simulink model "PubIfDecisionLSM_MDL"  (R2020b)
settings: configuration reference "DspaceConfig" (kept outside this file)
PostLoadFcn:
  | if any(exist('dsrtsu_mdlpostloadfcn', 'file') ~= 0), dsrtsu_mdlpostloadfcn('Execute', bdroot); end
InitFcn:
  | , if any(exist('rtifpga_mdlclblib', 'file') ~= 0), rtifpga_mdlclblib('Init', bdroot); end,
  | , if any(exist('dsmpb_private', 'file') ~= 0), dsmpb_private('dsmpb_mdlclblib', 'Init', bdroot); end,
values from neighbouring files (symbols this model uses):
  P_LSM_ALC_Enable = 0.0    [LSM_Parameter.sldd]
  P_LSM_AwayEdge_offset = 0.1    [LSM_Parameter.sldd]
  P_LSM_CentValidErr = 1.0    [LSM_Parameter.sldd]
  P_LSM_DOP_C0_EN_Limit = 0.8    [LSM_Parameter.sldd]
  P_LSM_DOP_C0_out_Limit = 2.0    [LSM_Parameter.sldd]
  P_LSM_DOP_C1_EN_Limit : value not decoded    [LSM_Parameter.sldd]
  P_LSM_DOP_C1_out_Limit : value not decoded    [LSM_Parameter.sldd]
  P_LSM_DOP_C1AndC2_Lim_X : value not decoded    [LSM_Parameter.sldd]
  P_LSM_DOP_C2_EN_Limit : value not decoded    [LSM_Parameter.sldd]
  P_LSM_DOP_C2_out_Limit : value not decoded    [LSM_Parameter.sldd]
  P_LSM_DOP_In_Pre2Dop_Dis = 1.0    [LSM_Parameter.sldd]
  P_LSM_DOP_Out_Pre2Dop_Dis = 2.0    [LSM_Parameter.sldd]
  P_LSM_DOP_PreDis_X : value not decoded    [LSM_Parameter.sldd]
  P_LSM_DOP_PreDis_Y : value not decoded    [LSM_Parameter.sldd]
  P_LSM_DOPEnableSW = 1.0    [LSM_Parameter.sldd]
  P_LSM_DOPValid_CheckTime = 0.06    [LSM_Parameter.sldd]
  P_LSM_DoubleLine_Curr2Cent_Dislimit = 0.5    [LSM_Parameter.sldd]
  P_LSM_DoubleLine_Dop2Cent_Dislimit = 0.5    [LSM_Parameter.sldd]
  P_LSM_DoubleLine_DOPOut_C1 : value not decoded    [LSM_Parameter.sldd]
  P_LSM_DoubleLine_Pre2Cent_Dislimit = 1.0    [LSM_Parameter.sldd]
  P_LSM_Error_Limit = 0.5    [LSM_Parameter.sldd]
  P_LSM_IFV2CenterAxis = 0.0    [LSM_Parameter.sldd]
  P_LSM_IFV2RearAxis = 0.0    [LSM_Parameter.sldd]
  P_LSM_Line2Edge_limit = 0.5    [LSM_Parameter.sldd]
  P_LSM_Line_Error = 0.1    [LSM_Parameter.sldd]
  P_LSM_LineSTD_Limit = 0.15    [LSM_Parameter.sldd]
  P_LSM_NOH_Switch = 0.0    [LSM_Parameter.sldd]
  P_LSM_OTL_C0_Factor = 1.0    [LSM_Parameter.sldd]
  P_LSM_OTL_C1_Factor = 0.5    [LSM_Parameter.sldd]
  P_LSM_OTL_C2_Factor = 0.5    [LSM_Parameter.sldd]
  P_LSM_Pre2OnlyLineDis = 5.0    [LSM_Parameter.sldd]
  P_LSM_Pre_t = 0.0    [LSM_Parameter.sldd]
  P_LSM_SingleLine_Cent2Edge_Dislimit = 100.0    [LSM_Parameter.sldd]
  P_LSM_SingleLine_Curr2Cent_Dislimit = 0.2    [LSM_Parameter.sldd]
  P_LSM_SingleLine_Dop2Cent_Dislimit = 0.2    [LSM_Parameter.sldd]
  P_LSM_SingleLine_DOPOut_C1 : value not decoded    [LSM_Parameter.sldd]
  P_LSM_SingleLine_Pre2Cent_Dislimit = 0.5    [LSM_Parameter.sldd]
  P_LSM_TJALimitSpd = 60.0    [LSM_Parameter.sldd]
undefined symbols (not defined in the file or in its folder): P_lCS_IFV2CenterAxis, P_LCS_IFV2RearAxis, P_LSM_EntryEdge_offset, P_LSM_EntryLnChngEnSwitch, P_LSM_EntryVanishDis, P_LSM_LinetLostTime, P_LSM_LineWijCal_C12, P_LSM_LineWijCal_C13, P_LSM_MapValid_ErrorSwitch, P_LSM_PosLineLcFac, P_LSM_SpdLim_Stub_Spd, P_LSM_SpdLim_StubLength, P_LSM_SpdTurnAlarm
libraries: simulink x324, TrueDurationTime x11
(part 16 of 25)

== stateflow chart PubIfDecisionLSM_MDL/Subsystem1/TargetLineCalc_20ms/TargetLineCalc/Subsystem3/Subsystem/Chart1 ==
  state on
    state CruiseValid2
      PilotRoadSts=18;
      LSM_PilotSPL=uint8(60);
      PilotSPLDist=uint16(0);
      state init
        state Name
          PilotTurnSwSts =0;
        state init4
          PilotTurnSwSts =6;
        state init5
          PilotTurnSwSts =3;
        state init3
          PilotTurnSwSts =7;
        (default) -> on.CruiseValid2.init.Name
        on.CruiseValid2.init.Name -> on.CruiseValid2.init.init3 [order 3] : [FrbRight>0]
        on.CruiseValid2.init.init3 -> on.CruiseValid2.init.Name : [FrbRight==0]
        on.CruiseValid2.init.Name -> on.CruiseValid2.init.init4 [order 1] : [FrbLeft>0]
        on.CruiseValid2.init.init4 -> on.CruiseValid2.init.Name : [FrbLeft==0]
        on.CruiseValid2.init.Name -> on.CruiseValid2.init.init5 [order 2] : [OneLane>0]
        on.CruiseValid2.init.init5 -> on.CruiseValid2.init.Name : [OneLane==0]
      state Name2
        PilotTurnSwSts=1;
      state init1
        PilotTurnSwSts =1;
      state init2
        PilotTurnSwSts =2;
      (default) -> on.CruiseValid2.init
      on.CruiseValid2.init -> on.CruiseValid2.Name2 [order 1] : [Vanish_turnleft>0]
      on.CruiseValid2.Name2 -> on.CruiseValid2.init : [Vanish_turnleft==0]
      on.CruiseValid2.init -> on.CruiseValid2.init1 [order 2] : [CruiseTurn>0&&...
          | TurnLeft>0]
      on.CruiseValid2.init1 -> on.CruiseValid2.init [order 1] : [CruiseTurn==0]
      on.CruiseValid2.init -> on.CruiseValid2.init2 [order 3] : [CruiseTurn>0&&...
          | TurnRight>0]
      on.CruiseValid2.init2 -> on.CruiseValid2.init [order 1] : [CruiseTurn==0]
      on.CruiseValid2.init2 -> on.CruiseValid2.init1 [order 2] : [TurnLeft>0]
      on.CruiseValid2.init1 -> on.CruiseValid2.init2 [order 2] : [TurnRight>0]
    state CruiseValid1
      PilotRoadSts=24;
      LSM_PilotSPL=0xff;
      PilotSPLDist=0xffff;
      state init
        state Name
          PilotTurnSwSts =0;
        state init4
          PilotTurnSwSts =6;
        state init5
          PilotTurnSwSts =3;
        state init3
          PilotTurnSwSts =7;
        (default) -> on.CruiseValid1.init.Name
        on.CruiseValid1.init.Name -> on.CruiseValid1.init.init3 [order 3] : [FrbRight>0]
        on.CruiseValid1.init.init3 -> on.CruiseValid1.init.Name : [FrbRight==0]
        on.CruiseValid1.init.Name -> on.CruiseValid1.init.init4 [order 1] : [FrbLeft>0]
        on.CruiseValid1.init.init4 -> on.CruiseValid1.init.Name : [FrbLeft==0]
        on.CruiseValid1.init.Name -> on.CruiseValid1.init.init5 [order 2] : [OneLane>0]
        on.CruiseValid1.init.init5 -> on.CruiseValid1.init.Name : [OneLane==0]
      state Name2
        PilotTurnSwSts=1;
      state init1
        PilotTurnSwSts =1;
      state init2
        PilotTurnSwSts =2;
      (default) -> on.CruiseValid1.init
      on.CruiseValid1.init -> on.CruiseValid1.Name2 [order 1] : [Vanish_turnleft>0]
      on.CruiseValid1.Name2 -> on.CruiseValid1.init : [Vanish_turnleft==0]
      on.CruiseValid1.init -> on.CruiseValid1.init1 [order 3] : [CruiseTurn>0&&...
          | TurnLeft>0]
      on.CruiseValid1.init1 -> on.CruiseValid1.init [order 1] : [CruiseTurn==0]
      on.CruiseValid1.init -> on.CruiseValid1.init2 [order 2] : [CruiseTurn>0&&...
          | TurnRight>0]
      on.CruiseValid1.init2 -> on.CruiseValid1.init [order 1] : [CruiseTurn==0]
      on.CruiseValid1.init2 -> on.CruiseValid1.init1 [order 2] : [TurnLeft>0]
      on.CruiseValid1.init1 -> on.CruiseValid1.init2 [order 2] : [TurnRight>0]
    state CruiseValid
      PilotRoadSts=17;
      LSM_PilotSPL=0xff;
      PilotSPLDist=0xffff;
      state init
        state Name
          PilotTurnSwSts =0;
        state init4
          PilotTurnSwSts =6;
        state init5
          PilotTurnSwSts =3;
        state init3
          PilotTurnSwSts =7;
        (default) -> on.CruiseValid.init.Name
        on.CruiseValid.init.Name -> on.CruiseValid.init.init3 [order 3] : [FrbRight>0]
        on.CruiseValid.init.init3 -> on.CruiseValid.init.Name : [FrbRight==0]
        on.CruiseValid.init.Name -> on.CruiseValid.init.init4 [order 1] : [FrbLeft>0]
        on.CruiseValid.init.init4 -> on.CruiseValid.init.Name : [FrbLeft==0]
        on.CruiseValid.init.Name -> on.CruiseValid.init.init5 [order 2] : [OneLane>0]
        on.CruiseValid.init.init5 -> on.CruiseValid.init.Name : [OneLane==0]
      state Name2
        PilotTurnSwSts=1;
      state init1
        PilotTurnSwSts =1;
      state init2
        PilotTurnSwSts =2;
      on.CruiseValid.init -> on.CruiseValid.Name2 [order 2] : [Vanish_turnleft>0]
      (default) -> on.CruiseValid.init
      on.CruiseValid.Name2 -> on.CruiseValid.init : [Vanish_turnleft==0]
      on.CruiseValid.init -> on.CruiseValid.init1 [order 1] : [CruiseTurn>0&&...
          | TurnLeft>0]
      on.CruiseValid.init1 -> on.CruiseValid.init [order 1] : [CruiseTurn==0]
      on.CruiseValid.init -> on.CruiseValid.init2 [order 3] : [CruiseTurn>0&&...
          | TurnRight>0]
      on.CruiseValid.init2 -> on.CruiseValid.init [order 1] : [CruiseTurn==0]
      on.CruiseValid.init2 -> on.CruiseValid.init1 [order 2] : [TurnLeft>0]
      on.CruiseValid.init1 -> on.CruiseValid.init2 [order 2] : [TurnRight>0]
    state EntryStub1
      PilotRoadSts=26;
      state Name
        PilotTurnSwSts =1;
      state Name1
        PilotTurnSwSts =4;
      (default) -> on.EntryStub1.Name
      on.EntryStub1.Name -> Name1 : [EntryStub5_TurnLeft==0]
      Name1 -> on.EntryStub1.Name : [EntryStub5_TurnLeft>0]
    state EntryStub2
      PilotTurnSwSts =0;
      PilotRoadSts=25;
    state StubValid
      state EntryStub3
        PilotTurnSwSts =4;
        PilotRoadSts=2;
      state EntryStub4
        PilotTurnSwSts =4;
        PilotRoadSts=1;
      state init
        PilotTurnSwSts =0;
        PilotRoadSts=0;
        LSM_PilotSPL=uint8(60);
        PilotSPLDist=uint16(f_distance);
      state EntryStub1
        PilotTurnSwSts =4;
        PilotRoadSts=2;
      state EntryStub2
        PilotTurnSwSts =4;
        PilotRoadSts=1;
      state Name
        PilotTurnSwSts =2;
        PilotRoadSts=7;
        LSM_PilotSPL=uint8(60);
        PilotSPLDist=uint16(f_distance);
      state LeftStub
        PilotTurnSwSts =1;
        PilotRoadSts=9;
        LSM_PilotSPL=uint8(60);
        PilotSPLDist=uint16(f_distance);
      state Name2
        PilotTurnSwSts =3;
        PilotRoadSts=7;
        LSM_PilotSPL=uint8(60);
        PilotSPLDist=uint16(f_distance);
      state Name3
        PilotTurnSwSts =5;
        PilotRoadSts=8;
        LSM_PilotSPL=uint8(60);
        PilotSPLDist=uint16(f_distance);
      state Name4
        PilotTurnSwSts =2;
        PilotRoadSts=20;
        LSM_PilotSPL=uint8(60);
        PilotSPLDist=uint16(f_distance);
      state CruiseLeft
        PilotTurnSwSts =3;
        PilotRoadSts=9;
        LSM_PilotSPL=uint8(60);
        PilotSPLDist=uint16(f_distance);
      state lExitStub3
        PilotTurnSwSts =1;
        PilotRoadSts=20;
        LSM_PilotSPL=uint8(60);
        PilotSPLDist=uint16(f_distance);
      state lExitStub1
        PilotTurnSwSts =5;
        PilotRoadSts=10;
        LSM_PilotSPL=uint8(60);
        PilotSPLDist=uint16(f_distance);
      state Name5
        PilotTurnSwSts =5;
        PilotRoadSts=19;
        LSM_PilotSPL=uint8(60);
        PilotSPLDist=uint16(f_distance);
      state lExitStub2
        PilotTurnSwSts =5;
        PilotRoadSts=19;
        LSM_PilotSPL=uint8(60);
        PilotSPLDist=uint16(f_distance);
      EntryStub4 -> EntryStub3 [order 1] : [EntryStub3>0]
      (default) -> on.StubValid.init
      EntryStub3 -> EntryStub4 [order 1] : [EntryStub4>0]
      on.StubValid.init -> EntryStub3 [order 2] : [EntryStub3>0]
      EntryStub3 -> on.StubValid.init [order 2] : [EntryStub3==0&&EntryStub4==0]
      on.StubValid.init -> EntryStub4 [order 4] : [EntryStub4>0]
      EntryStub4 -> on.StubValid.init [order 2] : [EntryStub3==0&&EntryStub4==0]
      on.StubValid.init -> on.StubValid.EntryStub1 [order 7] : [EntryStub1>0]
      on.StubValid.EntryStub1 -> on.StubValid.init [order 2] : [EntryStub1==0&&EntryStub2==0]
      on.StubValid.EntryStub1 -> on.StubValid.EntryStub2 [order 1] : [EntryStub2>0]
      on.StubValid.EntryStub2 -> on.StubValid.EntryStub1 [order 1] : [EntryStub1>0]
      on.StubValid.init -> on.StubValid.EntryStub2 [order 8] : [EntryStub2>0]
      on.StubValid.EntryStub2 -> on.StubValid.init [order 2] : [EntryStub1==0&&EntryStub2==0]
      (junction 434) -> on.StubValid.init
      (junction 453) -> on.StubValid.init
      on.StubValid.init -> CruiseLeft [order 5] : [CruiseLeft>0]
      CruiseLeft -> on.StubValid.init [order 3] : [CruiseLeft==0&&...
          | LeftStub==0&&...
          | rExitStub1==0]
      on.StubValid.init -> LeftStub [order 6] : [LeftStub>0]
      LeftStub -> on.StubValid.init [order 2] : [LeftStub==0&&CruiseLeft==0]
      on.StubValid.init -> lExitStub1 [order 10] : [lExitStub1>0]
      lExitStub3 -> on.StubValid.init [order 3] : [lExitStub2==0&&...
          | lExitStub3==0&&...
          | lExitStub1==0]
      (junction 266) -> on.StubValid.init
      (junction 280) -> on.StubValid.init
      on.StubValid.init -> on.StubValid.Name2 [order 3] : [CruiseRight>0]
      on.StubValid.Name2 -> on.StubValid.init [order 3] : [CruiseRight==0&&...
          | RightStub==0&&...
          | rExitStub1==0]
      on.StubValid.init -> on.StubValid.Name [order 1] : [RightStub>0]
      on.StubValid.Name -> on.StubValid.init [order 2] : [RightStub==0&&CruiseRight==0]
      on.StubValid.init -> Name3 [order 9] : [rExitStub1>0]
      Name4 -> on.StubValid.init [order 3] : [rExitStub2==0&&...
          | rExitStub3==0&&...
          | rExitStub1==0]
      on.StubValid.Name -> on.StubValid.Name2 [order 1] : [CruiseRight>0]
      LeftStub -> CruiseLeft [order 1] : [CruiseLeft>0]
      on.StubValid.Name2 -> on.StubValid.Name [order 2] : [RightStub>0]
      CruiseLeft -> LeftStub [order 2] : [LeftStub>0]
      on.StubValid.Name2 -> Name3 [order 1] : [rExitStub1>0]
      Name3 -> Name4 [order 1] : [rExitStub3>0]
      Name3 -> on.StubValid.Name2 [order 3] : [CruiseRight>0]
      CruiseLeft -> lExitStub1 [order 1] : [lExitStub1>0]
      lExitStub1 -> lExitStub3 [order 1] : [lExitStub3>0]
      lExitStub1 -> CruiseLeft [order 3] : [CruiseLeft>0]
      Name4 -> Name3 [order 2] : [rExitStub1>0]
      Name3 -> (junction 280) [order 4] : [CruiseRight==0&&...
          | rExitStub1==0&&...
          | rExitStub3==0&&...
          | rExitStub2==0]
      Name3 -> Name5 [order 2] : [rExitStub2>0]
      Name5 -> Name3 [order 2] : [rExitStub1>0]
      Name5 -> Name4 [order 1] : [rExitStub3>0]
      Name4 -> Name5 [order 1] : [rExitStub2>0]
      lExitStub3 -> lExitStub1 [order 2] : [lExitStub1>0]
      lExitStub1 -> (junction 453) [order 4] : [CruiseLeft==0&&...
          | lExitStub1==0&&...
          | lExitStub3==0&&...
          | lExitStub2==0]
      lExitStub3 -> lExitStub2 [order 1] : [lExitStub2>0]
      lExitStub2 -> lExitStub3 [order 1] : [lExitStub3>0]
      lExitStub1 -> lExitStub2 [order 2] : [lExitStub2>0]
      lExitStub2 -> lExitStub1 [order 2] : [lExitStub1>0]
      Name5 -> (junction 266) [order 3] : [rExitStub2==0&&rExitStub3==0&&rExitStub1==0]
      lExitStub2 -> (junction 434) [order 3] : [lExitStub2==0&&lExitStub3==0&&lExitStub1==0]
    (junction 533) -> (junction 532)
    CruiseValid -> (junction 533) [order 3] : [RoadType~=1&&RoadType~=2]
    (junction 532) -> CruiseValid2
    (junction 527) -> (junction 528)
    (junction 528) -> CruiseValid
    CruiseValid2 -> (junction 527) [order 1] : [RoadType==1]
    on.EntryStub1 -> CruiseValid [order 1] : [CruiseValid>0&&RoadType==1&&EntryStub5==0&&EntryStub6==0]
    CruiseValid -> on.EntryStub1 [order 4] : [EntryStub5>0]
    CruiseValid1 -> CruiseValid2 [order 3] : [RoadType~=1&&RoadType~=2]
    CruiseValid -> CruiseValid1 [order 2] : [RoadType==2]
    on.EntryStub2 -> on.EntryStub1 [order 2] : [EntryStub5>0]
    on.EntryStub1 -> on.EntryStub2 [order 2] : [EntryStub6>0]
    CruiseValid2 -> CruiseValid1 [order 3] : [RoadType==2]
    CruiseValid1 -> CruiseValid [order 2] : [RoadType==1]
    StubValid -> on.EntryStub1 [order 2] : [EntryStub5>0]
    on.EntryStub1 -> StubValid [order 3] : [EntryStub5==0&&EntryStub6==0]
    CruiseValid -> on.EntryStub2 [order 5] : [EntryStub6>0]
    on.EntryStub2 -> CruiseValid [order 1] : [CruiseValid>0&&...
        | RoadType==1&&...
        | EntryStub5==0&&...
        | EntryStub6==0]
    CruiseValid2 -> StubValid [order 2] : [StubValid>0]
    StubValid -> CruiseValid2 [order 5] : [CruiseValid>0&&RoadType~=1&&RoadType~=2&&EntryStub5==0&&EntryStub6==0]
    CruiseValid -> StubValid [order 1] : [StubValid>0]
    StubValid -> CruiseValid [order 1] : [CruiseValid>0&&RoadType==1&&EntryStub5==0&&EntryStub6==0]
    CruiseValid1 -> StubValid [order 1] : [StubValid>0]
    StubValid -> CruiseValid1 [order 4] : [CruiseValid>0&&RoadType==2&&EntryStub5==0&&EntryStub6==0]
    StubValid -> on.EntryStub2 [order 3] : [EntryStub6>0]
    on.EntryStub2 -> StubValid [order 3] : [EntryStub5==0&&EntryStub6==0]
    (default) -> StubValid
  state off1
    PilotTurnSwSts =0;
    PilotRoadSts =0;
    LSM_PilotSPL=0xff;
    PilotSPLDist=0xffff;
  (default) -> off1
  off1 -> on : [i_mapvalid==3&&i_on_nav_path>0]
  on -> off1 : [i_mapvalid~=3||i_on_nav_path==0]
  data: StubValid input boolean size=1; RightStub input boolean size=1; RoadType input uint8 size=1; PilotRoadSts output uint8 size=1; PilotTurnSwSts output uint8 size=1; LeftStub input boolean size=1; CruiseValid input boolean size=1; TurnLeft input boolean size=1; TurnRight input boolean size=1; Vanish_turnleft input boolean size=1; EntryStub1 input boolean size=1; rExitStub1 input boolean size=1; rExitStub2 input boolean size=1; i_mapvalid input uint8 size=1; i_on_nav_path input uint8 size=1; CruiseLeft input boolean size=1; CruiseRight input boolean size=1; f_distance input single size=1; LSM_PilotSPL output uint8 size=1; PilotSPLDist output uint16 size=1; CruiseTurn input boolean size=1; EntryStub2 input boolean size=1; lExitStub1 input boolean size=1; lExitStub2 input boolean size=1; lExitStub3 input boolean size=1; rExitStub3 input boolean size=1; FrbLeft input boolean size=1; FrbRight input boolean size=1; OneLane input boolean size=1; EntryStub3 input; EntryStub4 input; EntryStub5 input; EntryStub6 input; EntryStub5_TurnLeft input

== matlab function PubIfDecisionLSM_MDL/Subsystem1/TargetLineCalc_20ms/TargetLineCalc/Subsystem3/Subsystem/MATLAB Function ==
  data: NOH_Valid input boolean size=1; PilotSts output uint8 size=1; RoadType input uint8 size=1; rExitStub4_takeover input; lExitStub4_takeover input; EntryStub5_takeover input; Vanish_turnleft_takeover input
function PilotSts = fcn(NOH_Valid,RoadType,rExitStub4_takeover,lExitStub4_takeover,EntryStub5_takeover,Vanish_turnleft_takeover)
PilotSts=uint8(0);
if NOH_Valid == 1
    if RoadType == 1
        PilotSts = uint8(1); %NOH-HW Mode
    end
    if RoadType == 2
        PilotSts = uint8(4); %NOH-City Mode
    end
    if RoadType ~=1 && RoadType ~=2
        PilotSts = uint8(2); %NOH-Ramp Mode
    end
    if rExitStub4_takeover>0 || lExitStub4_takeover>0 || EntryStub5_takeover>0 || Vanish_turnleft_takeover>0
        PilotSts = uint8(3); %NOH-TakeOver
    end
end

== matlab function PubIfDecisionLSM_MDL/Subsystem1/TargetLineCalc_20ms/TargetLineCalc/Subsystem3/Subsystem2/MATLAB Function ==
  data: nLaneID input uint8 size=1; i_rec_lanes input uint8 size=8; Forbid_TurnRight output boolean size=1; Forbid_TurnLeft output boolean size=1; OneLane output boolean size=1; i_rec_lanes_num input
function [Forbid_TurnRight,Forbid_TurnLeft,OneLane] = fcn(nLaneID,i_rec_lanes,i_rec_lanes_num)

Forbid_TurnRight = false;
Forbid_TurnLeft = false;
OneLane = false;
m=uint8(1);
if i_rec_lanes_num == 1
    if nLaneID==i_rec_lanes(1)
        OneLane = true;
    end
end
if i_rec_lanes_num > 1 
    if i_rec_lanes(1)>1 && nLaneID==i_rec_lanes(1)
        Forbid_TurnLeft = true;
    end

    for i=uint8(1):length(i_rec_lanes)
        if i_rec_lanes(i)>0
            m=i;
        end
    end

    if nLaneID == i_rec_lanes(m)
        Forbid_TurnRight = true;
    end
end

== matlab function PubIfDecisionLSM_MDL/Subsystem1/TargetLineCalc_20ms/TargetLineCalc/Subsystem3/Subsystem2/Subsystem/MATLAB Function14 ==
  data: u input; y output; i_k input; i output uint8
function [y,i] = fcn(u,i_k)
y = uint8(0);
i = i_k;
if u>2 || u<-2
    i = i+1;
else
    i = uint8(0);
end
if i>10
    y = uint8(1);
end

== matlab function PubIfDecisionLSM_MDL/Subsystem1/TargetLineCalc_20ms/TargetLineCalc/Subsystem3/Subsystem2/Subsystem1/MATLAB Function14 ==
  data: u input; y output; i_k input; i output uint8
function [y,i] = fcn(u,i_k)
y = uint8(0);
i = i_k;
if u>2 || u<-2
    i = i+1;
else
    i = uint8(0);
end
if i>10
    y = uint8(1);
end

== matlab function PubIfDecisionLSM_MDL/Subsystem1/TargetLineCalc_20ms/TargetLineCalc/Subsystem3/Subsystem2/Subsystem10/MATLAB Function14 ==
  data: u input; y output; i_k input; i output uint8
function [y,i] = fcn(u,i_k)
y = uint8(0);
i = i_k;
if u>2 || u<-2
    i = i+1;
else
    i = uint8(0);
end
if i>10
    y = uint8(1);
end

== matlab function PubIfDecisionLSM_MDL/Subsystem1/TargetLineCalc_20ms/TargetLineCalc/Subsystem2/MATLAB Function ==
  data: TJA_Line input; DOP_CO input; DOP_C1 input; DOP_C2 input; DOP_CO_EN_Limit input; DOP_C1_EN_Limit input; DOP_C2_EN_Limit input; DOP_CO_out_Limit input; DOP_C1_out_Limit input; DOP_C2_out_Limit input; DOP_In_Pre2Dop_Dis input; DOP_Out_Pre2Dop_Dis input; DOP_Valid input; dy_pre input; Y_DOP input; DOP_In_Enable output boolean; DOP_Out_Enable output
function [DOP_In_Enable,DOP_Out_Enable] = fcn(TJA_Line,DOP_CO,DOP_C1,DOP_C2,DOP_CO_EN_Limit,DOP_C1_EN_Limit,...
    DOP_C2_EN_Limit,DOP_CO_out_Limit,DOP_C1_out_Limit,DOP_C2_out_Limit,DOP_In_Pre2Dop_Dis,DOP_Out_Pre2Dop_Dis,DOP_Valid,dy_pre,Y_DOP)
DOP_In_Enable = false;
DOP_Out_Enable = false;
if TJA_Line~=2 && DOP_Valid>0
    if abs(DOP_CO)<DOP_CO_EN_Limit&&...
            abs(DOP_C1)<DOP_C1_EN_Limit&&...
            abs(DOP_C2)<DOP_C2_EN_Limit&&...
            abs(dy_pre-Y_DOP)<DOP_In_Pre2Dop_Dis
        
        DOP_In_Enable = true;
        
    end
elseif TJA_Line==2
     if abs(DOP_CO)>DOP_CO_out_Limit||...
             abs(DOP_C1)>DOP_C1_out_Limit||...
             abs(DOP_C2)>DOP_C2_out_Limit||...
             abs(dy_pre-Y_DOP)>DOP_Out_Pre2Dop_Dis||...
             DOP_Valid==0
         
        DOP_Out_Enable = true;
        
     end
end

== matlab function PubIfDecisionLSM_MDL/Subsystem1/TargetLineCalc_20ms/TargetLineCalc/Subsystem3/Subsystem2/Subsystem11/MATLAB Function14 ==
  data: u input; y output; i_k input; i output uint8
function [y,i] = fcn(u,i_k)
y = uint8(0);
i = i_k;
if u>2 || u<-2
    i = i+1;
else
    i = uint8(0);
end
if i>10
    y = uint8(1);
end

== matlab function PubIfDecisionLSM_MDL/Subsystem1/TargetLineCalc_20ms/TargetLineCalc/Subsystem3/Subsystem2/Subsystem12/MATLAB Function14 ==
  data: u input; y output; i_k input; i output uint8
function [y,i] = fcn(u,i_k)
y = uint8(0);
i = i_k;
if u>2 || u<-2
    i = i+1;
else
    i = uint8(0);
end
if i>10
    y = uint8(1);
end

== matlab function PubIfDecisionLSM_MDL/Subsystem1/TargetLineCalc_20ms2/LALine ==
  data: LA_Count input; L1Conf output uint8 size=1; L1C0 output single size=1; L1C1 output single size=1; L1C2 output single size=1; L1C3 output single size=1; L1DxMin output single size=1; L1DxMax output single size=1; L1A0 input single size=1; L1A1 input single size=1; L1A2 input single size=1; L1A3 input single size=1; L1RaMin input single size=1; L1RaMax input single size=1; L1Avail input uint8 size=1; L1LineType input uint8 size=1; L1DLType input uint8 size=1; L1SideType input uint8 size=1; L1Wid input single size=1; L1Confidence input; L2A0 input single size=1; L2A1 input single size=1; L2A2 input single size=1; L2A3 input single size=1; L2RaMin input single size=1; L2RaMax input single size=1; L2Avail input uint8 size=1; L2LineType input uint8 size=1; L2DLType input uint8 size=1; L2SideType input uint8 size=1; L2Wid input single size=1; L2Confidence input; L3A0 input single size=1; L3A1 input single size=1; L3A2 input single size=1; L3A3 input single size=1; L3RaMin input single size=1; L3RaMax input single size=1; L3Avail input uint8 size=1; L3LineType input uint8 size=1; L3DLType input uint8 size=1; L3SideType input uint8 size=1; L3Wid input single size=1; L3Confidence input; L4A0 input single size=1; L4A1 input single size=1; L4A2 input single size=1; L4A3 input single size=1; L4RaMin input single size=1; L4RaMax input single size=1; L4Avail input uint8 size=1; L4LineType input uint8 size=1; L4DLType input uint8 size=1; L4SideType input uint8 size=1; L4Wid input single size=1; L1Type output uint8 size=1; L1DLM output uint8 size=1; L1Width output single size=1; L1Reliable output; L2Conf output uint8 size=1; L2C0 output single size=1; L2C1 output single size=1; L2C2 output single size=1; L2C3 output single size=1; L2DxMin output single size=1; L2DxMax output single size=1; L2Type output uint8 size=1; L2DLM output uint8 size=1; L2Width output single size=1; L2Reliable output; L3Conf output uint8 size=1; L3C0 output single size=1; L3C1 output single size=1; L3C2 output single size=1; L3C3 output single size=1; L3DxMin output single size=1; L3DxMax output single size=1; L3Type output uint8 size=1; L3DLM output uint8 size=1; L3Width output single size=1; L3Reliable output; L4Conf output uint8 size=1; L4C0 output single size=1; L4C1 output single size=1; L4C2 output single size=1; L4C3 output single size=1; L4DxMin output single size=1; L4DxMax output single size=1; L4Type output uint8 size=1; L4DLM output uint8 size=1; L4Width output single size=1; L4Confidence input; L4Reliable output
function [L1Conf,L1C0,L1C1,L1C2,L1C3,L1DxMin,L1DxMax,L1Type,L1DLM,L1Width,L1Reliable,...
    L2Conf,L2C0,L2C1,L2C2,L2C3,L2DxMin,L2DxMax,L2Type,L2DLM,L2Width,L2Reliable,...
    L3Conf,L3C0,L3C1,L3C2,L3C3,L3DxMin,L3DxMax,L3Type,L3DLM,L3Width,L3Reliable,...
    L4Conf,L4C0,L4C1,L4C2,L4C3,L4DxMin,L4DxMax,L4Type,L4DLM,L4Width,L4Reliable]...
    = LA(LA_Count,L1A0,L1A1,L1A2,L1A3,L1RaMin,L1RaMax,L1Avail,L1LineType,L1DLType,L1SideType,L1Wid,L1Confidence,...
    L2A0,L2A1,L2A2,L2A3,L2RaMin,L2RaMax,L2Avail,L2LineType,L2DLType,L2SideType,L2Wid,L2Confidence,...
    L3A0,L3A1,L3A2,L3A3,L3RaMin,L3RaMax,L3Avail,L3LineType,L3DLType,L3SideType,L3Wid,L3Confidence,...
    L4A0,L4A1,L4A2,L4A3,L4RaMin,L4RaMax,L4Avail,L4LineType,L4DLType,L4SideType,L4Wid,L4Confidence)

L1Conf = uint8(0);
L1C0 = single(0);
L1C1 = single(0);
L1C2 = single(0);
L1C3 = single(0);
L1DxMin = single(0);
L1DxMax = single(0);
L1Type = uint8(0);
L1DLM = uint8(0);
L1Width = single(0);
L1Reliable = single(0);

L2Conf = uint8(0);
L2C0 = single(0);
L2C1 = single(0);
L2C2 = single(0);
L2C3 = single(0);
L2DxMin = single(0);
L2DxMax = single(0);
L2Type = uint8(0);
L2DLM = uint8(0);
L2Width = single(0);
L2Reliable = single(0);

L3Conf = uint8(0);
L3C0 = single(0);
L3C1 = single(0);
L3C2 = single(0);
L3C3 = single(0);
L3DxMin = single(0);
L3DxMax = single(0);
L3Type = uint8(0);
L3DLM = uint8(0);
L3Width = single(0);
L3Reliable = single(0);

L4Conf = uint8(0);
L4C0 = single(0);
L4C1 = single(0);
L4C2 = single(0);
L4C3 = single(0);
L4DxMin = single(0);
L4DxMax = single(0);
L4Type = uint8(0);
L4DLM = uint8(0);
L4Width = single(0);
L4Reliable = single(0);
%%  临车道车道线预处理
if LA_Count >= 1                                     %临车道车道线数量
    if L1SideType==1                                 %左左车道线
        L1Conf = L1Avail;
        L1C0 = L1A0;
        L1C1 = L1A1;
        L1C2 = L1A2;
        L1C3 = L1A3;
        L1DxMin = L1RaMin;
        L1DxMax = L1RaMax;
        L1Type = L1LineType;
        L1DLM = L1DLType;
        L1Width = L1Wid;
        L1Reliable = L1Confidence;
    elseif L1SideType==2                             %左车道右侧车道线
        L2Conf = L1Avail;
        L2C0 = L1A0;
        L2C1 = L1A1;
        L2C2 = L1A2;
        L2C3 = L1A3;
        L2DxMin = L1RaMin;
        L2DxMax = L1RaMax;
        L2Type = L1LineType;
        L2DLM = L1DLType;
        L2Width = L1Wid;
        L2Reliable = L1Confidence;
    elseif L1SideType==3                             %右车道左侧车道线
        L3Conf = L1Avail;
        L3C0 = L1A0;
        L3C1 = L1A1;
        L3C2 = L1A2;
        L3C3 = L1A3;
        L3DxMin = L1RaMin;
        L3DxMax = L1RaMax;
        L3Type = L1LineType;
        L3DLM = L1DLType;
        L3Width = L1Wid;
        L3Reliable = L1Confidence;
    elseif L1SideType==4                             %右右车道线
        L4Conf = L1Avail;
        L4C0 = L1A0;
        L4C1 = L1A1;
        L4C2 = L1A2;
        L4C3 = L1A3;
        L4DxMin = L1RaMin;
        L4DxMax = L1RaMax;
        L4Type = L1LineType;
        L4DLM = L1DLType;
        L4Width = L1Wid;
        L4Reliable = L1Confidence;
    end
    if LA_Count >= 2
        if L2SideType==1
            L1Conf = L2Avail;
            L1C0 = L2A0;
            L1C1 = L2A1;
            L1C2 = L2A2;
            L1C3 = L2A3;
            L1DxMin = L2RaMin;
            L1DxMax = L2RaMax;
            L1Type = L2LineType;
            L1DLM = L2DLType;
            L1Width = L2Wid;
            L1Reliable = L2Confidence;
        elseif L2SideType==2
            L2Conf = L2Avail;
            L2C0 = L2A0;
            L2C1 = L2A1;
            L2C2 = L2A2;
            L2C3 = L2A3;
            L2DxMin = L2RaMin;
            L2DxMax = L2RaMax;
            L2Type = L2LineType;
            L2DLM = L2DLType;
            L2Width = L2Wid;
            L2Reliable = L2Confidence;
        elseif L2SideType==3
            L3Conf = L2Avail;
            L3C0 = L2A0;
            L3C1 = L2A1;
            L3C2 = L2A2;
            L3C3 = L2A3;
            L3DxMin = L2RaMin;
            L3DxMax = L2RaMax;
            L3Type = L2LineType;
            L3DLM = L2DLType;
            L3Width = L2Wid;
            L3Reliable = L2Confidence;
        elseif L2SideType==4
            L4Conf = L2Avail;
            L4C0 = L2A0;
            L4C1 = L2A1;
            L4C2 = L2A2;
            L4C3 = L2A3;
            L4DxMin = L2RaMin;
            L4DxMax = L2RaMax;
            L4Type = L2LineType;
            L4DLM = L2DLType;
            L4Width = L2Wid;
            L4Reliable = L2Confidence;
        end
        if LA_Count >= 3
            if L3SideType==1
                L1Conf = L3Avail;
                L1C0 = L3A0;
                L1C1 = L3A1;
                L1C2 = L3A2;
                L1C3 = L3A3;
                L1DxMin = L3RaMin;
                L1DxMax = L3RaMax;
                L1Type = L3LineType;
                L1DLM = L3DLType;
                L1Width = L3Wid;
                L1Reliable = L3Confidence;
            elseif L3SideType==2
                L2Conf = L3Avail;
                L2C0 = L3A0;
                L2C1 = L3A1;
                L2C2 = L3A2;
                L2C3 = L3A3;
                L2DxMin = L3RaMin;
                L2DxMax = L3RaMax;
                L2Type = L3LineType;
                L2DLM = L3DLType;
                L2Width = L3Wid;
                L2Reliable = L3Confidence;
            elseif L3SideType==3
                L3Conf = L3Avail;
                L3C0 = L3A0;
                L3C1 = L3A1;
                L3C2 = L3A2;
                L3C3 = L3A3;
                L3DxMin = L3RaMin;
                L3DxMax = L3RaMax;
                L3Type = L3LineType;
                L3DLM = L3DLType;
                L3Width = L3Wid;
                L3Reliable = L3Confidence;
            elseif L3SideType==4
                L4Conf = L3Avail;
                L4C0 = L3A0;
                L4C1 = L3A1;
                L4C2 = L3A2;
                L4C3 = L3A3;
                L4DxMin = L3RaMin;
                L4DxMax = L3RaMax;
                L4Type = L3LineType;
                L4DLM = L3DLType;
                L4Width = L3Wid;
                L4Reliable = L3Confidence;
            end
            if LA_Count >= 4
                if L4SideType==1
                    L1Conf = L4Avail;
                    L1C0 = L4A0;
                    L1C1 = L4A1;
                    L1C2 = L4A2;
                    L1C3 = L4A3;
                    L1DxMin = L4RaMin;
                    L1DxMax = L4RaMax;
                    L1Type = L4LineType;
                    L1DLM = L4DLType;
                    L1Width = L4Wid;
                    L1Reliable = L4Confidence;
                elseif L4SideType==2
                    L2Conf = L4Avail;
                    L2C0 = L4A0;
                    L2C1 = L4A1;
                    L2C2 = L4A2;
                    L2C3 = L4A3;
                    L2DxMin = L4RaMin;
                    L2DxMax = L4RaMax;
                    L2Type = L4LineType;
                    L2DLM = L4DLType;
                    L2Width = L4Wid;
                    L2Reliable = L4Confidence;
                elseif L4SideType==3
                    L3Conf = L4Avail;
                    L3C0 = L4A0;
                    L3C1 = L4A1;
                    L3C2 = L4A2;
                    L3C3 = L4A3;
                    L3DxMin = L4RaMin;
                    L3DxMax = L4RaMax;
                    L3Type = L4LineType;
                    L3DLM = L4DLType;
                    L3Width = L4Wid;
                    L3Reliable = L4Confidence;
                elseif L4SideType==4
                    L4Conf = L4Avail;
                    L4C0 = L4A0;
                    L4C1 = L4A1;
                    L4C2 = L4A2;
                    L4C3 = L4A3;
                    L4DxMin = L4RaMin;
                    L4DxMax = L4RaMax;
                    L4Type = L4LineType;
                    L4DLM = L4DLType;
                    L4Width = L4Wid;
                    L4Reliable = L4Confidence;
                end
            end
        end
    end
end

== stateflow chart PubIfDecisionLSM_MDL/Subsystem1/TargetLineCalc_20ms/TargetLineCalc/Subsystem2/TJA_Line_Select ==
  state OFF
    en:
    TJA_Line = uint8(0);
    TJA_Source = uint8(0);
  state DOP_Line
    en:
    TJA_Line = uint8(2);
    TJA_Source = uint8(1);
  state EQ4_Line
    en:
    TJA_Line = uint8(1);
    TJA_Source = uint8(0);
  (default) -> OFF
  OFF -> DOP_Line [order 2] : [Off2DOP_flag]
  OFF -> EQ4_Line [order 1] : [Off2Cent_flag]
  DOP_Line -> OFF [order 2] : [DOP2Off_flag]
  EQ4_Line -> OFF [order 2] : [Cent2Off_flag]
  EQ4_Line -> DOP_Line [order 1] : [Cent2DOP_flag]
  DOP_Line -> EQ4_Line [order 1] : [DOP2Cent_flag]
  data: TJA_Line output uint8 size=1; Cent2Off_flag input uint8 size=1; DOP2Cent_flag input uint8 size=1; DOP2Off_flag input uint8 size=1; Off2Cent_flag input uint8 size=1; Off2DOP_flag input uint8 size=1; Cent2DOP_flag input uint8 size=1; TJA_Source output uint8 size=1

== matlab function PubIfDecisionLSM_MDL/Subsystem1/TargetLineCalc_20ms/TargetLineCalc/Subsystem3/Subsystem2/Subsystem13/MATLAB Function14 ==
  data: u input; y output; i_k input; i output uint8
function [y,i] = fcn(u,i_k)
y = uint8(0);
i = i_k;
if u>2 || u<-2
    i = i+1;
else
    i = uint8(0);
end
if i>10
    y = uint8(1);
end

== matlab function PubIfDecisionLSM_MDL/Subsystem1/TargetLineCalc_20ms/TargetLineCalc/Subsystem3/Subsystem2/Subsystem14/MATLAB Function14 ==
  data: u input; y output; i_k input; i output uint8
function [y,i] = fcn(u,i_k)
y = uint8(0);
i = i_k;
if u>2 || u<-2
    i = i+1;
else
    i = uint8(0);
end
if i>10
    y = uint8(1);
end

== matlab function PubIfDecisionLSM_MDL/Subsystem1/TargetLineCalc_20ms/TargetLineCalc/Subsystem3/Subsystem2/Subsystem15/MATLAB Function14 ==
  data: u input; y output; i_k input; i output uint8
function [y,i] = fcn(u,i_k)
y = uint8(0);
i = i_k;
if u>2 || u<-2
    i = i+1;
else
    i = uint8(0);
end
if i>10
    y = uint8(1);
end

== matlab function PubIfDecisionLSM_MDL/Subsystem1/TargetLineCalc_20ms/TargetLineCalc/Subsystem3/Subsystem2/Subsystem16/MATLAB Function14 ==
  data: u input; y output; i_k input; i output uint8
function [y,i] = fcn(u,i_k)
y = uint8(0);
i = i_k;
if u>2 || u<-2
    i = i+1;
else
    i = uint8(0);
end
if i>10
    y = uint8(1);
end

== matlab function PubIfDecisionLSM_MDL/Subsystem1/TargetLineCalc_20ms/TargetLineCalc/Subsystem3/Subsystem2/Subsystem2/MATLAB Function14 ==
  data: u input; y output; i_k input; i output uint8
function [y,i] = fcn(u,i_k)
y = uint8(0);
i = i_k;
if u>2 || u<-2
    i = i+1;
else
    i = uint8(0);
end
if i>10
    y = uint8(1);
end

== matlab function PubIfDecisionLSM_MDL/Subsystem1/TargetLineCalc_20ms/TargetLineCalc/Subsystem3/Subsystem2/Subsystem3/MATLAB Function14 ==
  data: u input; y output; i_k input; i output uint8
function [y,i] = fcn(u,i_k)
y = uint8(0);
i = i_k;
if u>2 || u<-2
    i = i+1;
else
    i = uint8(0);
end
if i>10
    y = uint8(1);
end

== matlab function PubIfDecisionLSM_MDL/Subsystem1/TargetLineCalc_20ms/TargetLineCalc/Subsystem3/Subsystem2/Subsystem4/MATLAB Function14 ==
  data: u input; y output; i_k input; i output uint8
function [y,i] = fcn(u,i_k)
y = uint8(0);
i = i_k;
if u>2 || u<-2
    i = i+1;
else
    i = uint8(0);
end
if i>10
    y = uint8(1);
end

== matlab function PubIfDecisionLSM_MDL/Subsystem1/TargetLineCalc_20ms/TargetLineCalc/Subsystem3/Subsystem2/Subsystem5/MATLAB Function14 ==
  data: u input; y output; i_k input; i output uint8
function [y,i] = fcn(u,i_k)
y = uint8(0);
i = i_k;
if u>2 || u<-2
    i = i+1;
else
    i = uint8(0);
end
if i>10
    y = uint8(1);
end

== matlab function PubIfDecisionLSM_MDL/Subsystem1/TargetLineCalc_20ms/TargetLineCalc/Subsystem3/Subsystem2/Subsystem6/MATLAB Function14 ==
  data: u input; y output; i_k input; i output uint8
function [y,i] = fcn(u,i_k)
y = uint8(0);
i = i_k;
if u>2 || u<-2
    i = i+1;
else
    i = uint8(0);
end
if i>10
    y = uint8(1);
end

== matlab function PubIfDecisionLSM_MDL/Subsystem1/TargetLineCalc_20ms/TargetLineCalc/Subsystem3/Subsystem2/Subsystem7/MATLAB Function14 ==
  data: u input; y output; i_k input; i output uint8
function [y,i] = fcn(u,i_k)
y = uint8(0);
i = i_k;
if u>2 || u<-2
    i = i+1;
else
    i = uint8(0);
end
if i>10
    y = uint8(1);
end

== matlab function PubIfDecisionLSM_MDL/Subsystem1/TargetLineCalc_20ms/TargetLineCalc/Subsystem3/Subsystem2/Subsystem8/MATLAB Function14 ==
  data: u input; y output; i_k input; i output uint8
function [y,i] = fcn(u,i_k)
y = uint8(0);
i = i_k;
if u>2 || u<-2
    i = i+1;
else
    i = uint8(0);
end
if i>10
    y = uint8(1);
end

== matlab function PubIfDecisionLSM_MDL/Subsystem1/TargetLineCalc_20ms/TargetLineCalc/Subsystem3/Subsystem2/Subsystem9/MATLAB Function14 ==
  data: u input; y output; i_k input; i output uint8
function [y,i] = fcn(u,i_k)
y = uint8(0);
i = i_k;
if u>2 || u<-2
    i = i+1;
else
    i = uint8(0);
end
if i>10
    y = uint8(1);
end

== matlab function PubIfDecisionLSM_MDL/Subsystem1/TargetLineCalc_20ms/TargetLineCalc/Subsystem4/MATLAB Function2 ==
  data: HWASts input; Changelane output; HWAStsK1 input; Lock_counterK1 input uint8; Lock_counter output
function [Changelane,Lock_counter]  = fcn(HWASts,HWAStsK1,Lock_counterK1)
Lock_counter = max(Lock_counterK1-uint8(1),uint8(0));
Changelane = uint8(0);
if HWASts == 5 || HWASts == 6
    Changelane = uint8(1);
elseif HWASts==3
    if HWAStsK1==5 || HWAStsK1==6 ||HWAStsK1==1 || HWAStsK1==2
        Lock_counter = uint8(250);
    end
    if Lock_counter>0
        Changelane = uint8(1);
    end
end

== matlab function PubIfDecisionLSM_MDL/Subsystem1/TargetLineCalc_20ms/TargetLineCalc/Subsystem4/MATLAB Function3 ==
  data: C12 input; Fac1 output single; C13 input; Fac2 output single; Fac3 output single
function [Fac1,Fac2,Fac3]  = fcn(C12,C13)

C21 = 1/C12;
C31 = 1/C13;

C32 = C12/C13;

C23 = C13/C12;



C = [1,   C12,   C13;
    C21,   1,    C23;
    C31,  C32,    1];

Fac1 = 1/(1 + C21 + C31 );
Fac2 = 1/(C12 + 1+ C32 );
Fac3 = 1/(C13 + C23 + 1 );

== matlab function PubIfDecisionLSM_MDL/Subsystem1/TargetLineCalc_20ms/TargetLineCalc/Subsystem4/MATLAB Function6 ==
  data: kap input; preDis input; CentLineValidK1 input; CentLineC3K1 input; CentLineC2K1 input; CentLineC1K1 input; CentLineC0K1 input; VisLineA3 input; VisLineA2 input; VisLineA1 input; VisLineA0 input; n1 input; n2 input; CosOfPsi input; SinOfPsi input; dDeltaX input; dDeltaY input; d_cur2 output; delta_d2 output; d_cur3 output; delta_d3 output; HWASts input
function [d_cur2,delta_d2,d_cur3,delta_d3] = ...
    fcn( kap,preDis,CentLineValidK1,CentLineC3K1,CentLineC2K1,CentLineC1K1,CentLineC0K1,...
    VisLineA3,VisLineA2,VisLineA1,VisLineA0,n1,n2,...
    CosOfPsi,SinOfPsi,dDeltaX,dDeltaY,HWASts)

xi = [single(1);single(2);single(3);single(4)];
yi = CentLineC3K1*xi.^3 + CentLineC2K1*xi.^2 + CentLineC1K1*xi + CentLineC0K1;
t_dx = xi-dDeltaX;
t_dy = yi-dDeltaY;
TmpX = t_dx*CosOfPsi+t_dy*SinOfPsi;
TmpY = -t_dx*SinOfPsi+t_dy*CosOfPsi;
[t3,t2,t1,t0] = pl(TmpX,TmpY);

if CentLineValidK1
    m1 = n1;
    m2 = n2;
else
    m1 = single(0);
    m2 = single(0);
end


RefA3_2 = t3*m1;
RefA2_2 = t2*m1 + (1-m1)*(0.5*kap);
RefA1_2 = t1*m1;
RefA0_2 = t0*m1;

RefA3_3 = t3*m2;
RefA2_3 = t2*m2 + (1-m2)*(0.5*kap);
RefA1_3 = t1*m2;
RefA0_3 = t0*m2;

y2 = RefA3_2*(preDis^3) + RefA2_2*(preDis^2) + RefA1_2*preDis + RefA0_2;
y3 = RefA3_3*(preDis^3) + RefA2_3*(preDis^2) + RefA1_3*preDis + RefA0_3;

if HWASts == 5 || HWASts == 6
    d_cur2 = abs(VisLineA0(2) - RefA0_2);
    d_cur3 = abs(RefA0_3 - VisLineA0(3));
else
    d_cur2 = VisLineA0(2) - RefA0_2;
    d_cur3 = RefA0_3 - VisLineA0(3);
end


d_pre2 = abs((VisLineA0(2) + VisLineA1(2)*preDis + VisLineA2(2)*(preDis^2) + VisLineA3(2)*(preDis^3)) - y2);  %预瞄点的距离
d_pre3 = abs((VisLineA0(3) + VisLineA1(3)*preDis + VisLineA2(3)*(preDis^2) + VisLineA3(3)*(preDis^3)) - y3);
delta_d2 = abs(d_pre2 - d_cur2);
delta_d3 = abs(d_pre3 - d_cur3);

== matlab function PubIfDecisionLSM_MDL/Subsystem1/TargetLineCalc_20ms/TargetLineCalc/Subsystem4/MATLAB Function7 ==
  data: dy2_Ran output; L2_R input; dy3_Ran output; L3_R input
function [dy2_Ran,dy3_Ran] = fcn(L2_R,L3_R)
dy2_Ran = L2_R;
dy3_Ran= L3_R;

== matlab function PubIfDecisionLSM_MDL/Subsystem1/TargetLineCalc_20ms/TargetLineCalc/Subsystem4/MATLAB Function8 ==
  data: VisLineReliable input; dy2_Rel output; dy3_Rel output
function [dy2_Rel,dy3_Rel] = fcn(VisLineReliable)
dy2_Rel = VisLineReliable(2);
dy3_Rel = VisLineReliable(3);

== matlab function PubIfDecisionLSM_MDL/Subsystem1/TargetLineCalc_20ms/TargetLineCalc/Subsystem5/MATLAB Function2 ==
  data: HWASts input; Changelane output; HWAStsK1 input; Lock_counterK1 input uint8; Lock_counter output
function [Changelane,Lock_counter]  = fcn(HWASts,HWAStsK1,Lock_counterK1)
Lock_counter = max(Lock_counterK1-uint8(1),uint8(0));
Changelane = uint8(0);
if HWASts == 5 || HWASts == 6
    Changelane = uint8(1);
elseif HWASts==3
    if HWAStsK1==5 || HWAStsK1==6 ||HWAStsK1==1 || HWAStsK1==2
        Lock_counter = uint8(250);
    end
    if Lock_counter>0
        Changelane = uint8(1);
    end
end

== matlab function PubIfDecisionLSM_MDL/Subsystem1/TargetLineCalc_20ms/TargetLineCalc/Subsystem2/LineSelect1 ==
  data: Off2Cent_flag output; Off2DOP_flag output; Cent2Off_flag output; DOP2Off_flag output; Cent2DOP_flag output; DOP2Cent_flag output; dy_pre output; Y_DOP output; Pre_dis input single; Line_State input; kap input single size=1; LCKSts input; CentLaneValid input boolean size=1; CentLineA3 input single size=1; CentLineA2 input single size=1; CentLineA1 input single size=1; CentLineA0 input single size=1; CentRange input single size=1; aOTL input single size=1; bOTL input single size=1; cOTL input single size=1; dOTL input single size=1; VisEdgeConf input uint8; VisEdgeA3 input single size=2; VisEdgeA2 input single size=2; VisEdgeA1 input single size=2; VisEdgeA0 input single size=2; DoubleLine_Pre2Cent_Dislimit input; DoubleLine_Curr2Cent_Dislimit input; DoubleLine_Dop2Cent_Dislimit input; SingleLine_Cent2Edge_Dislimit input; SingleLine_Pre2Cent_Dislimit input; SingleLine_Curr2Cent_Dislimit input; SingleLine_Dop2Cent_Dislimit input; SingleLine_DOPOut_C1 input; DoubleLine_DOPOut_C1 input; Vehicle_Speed input; DOP_EN input boolean; DOP_OUT input boolean
function [Off2Cent_flag,Off2DOP_flag,Cent2Off_flag,DOP2Off_flag,Cent2DOP_flag,DOP2Cent_flag,dy_pre,Y_DOP]= ...
    LineSelect(Pre_dis,Line_State,kap,LCKSts,...
    CentLaneValid,CentLineA3,CentLineA2,CentLineA1,CentLineA0,CentRange,...
    aOTL,bOTL,cOTL,dOTL,...
    VisEdgeConf,VisEdgeA3,VisEdgeA2,VisEdgeA1,VisEdgeA0,...
    DoubleLine_Pre2Cent_Dislimit,DoubleLine_Curr2Cent_Dislimit,DoubleLine_Dop2Cent_Dislimit,...
    SingleLine_Cent2Edge_Dislimit,SingleLine_Pre2Cent_Dislimit,SingleLine_Curr2Cent_Dislimit,SingleLine_Dop2Cent_Dislimit,...
    SingleLine_DOPOut_C1,DoubleLine_DOPOut_C1,...
    Vehicle_Speed,DOP_EN,DOP_OUT)

DOP2Cent_flag = uint8(0);
Off2Cent_flag=uint8(0);
Off2DOP_flag=uint8(0);
Cent2Off_flag=uint8(0);
DOP2Off_flag=uint8(0);
Cent2DOP_flag=uint8(0);

dy_pre = 0.5*kap*Pre_dis^2;

% CuratureCent_pre = CentLineA1 + 2*CentLineA2*preDis + 3*CentLineA3*(preDis^2);
CuratureDop_pre = cOTL + 2*bOTL*Pre_dis + 3*aOTL*(Pre_dis^2);
Y_Line = CentLineA0+CentLineA1*Pre_dis+CentLineA2*Pre_dis^2+CentLineA3*Pre_dis^3;
Y_DOP = dOTL+cOTL*Pre_dis+bOTL*Pre_dis^2+aOTL*Pre_dis^3;
dyLeRE = (VisEdgeA0(1) + VisEdgeA1(1)*Pre_dis + VisEdgeA2(1)*(Pre_dis^2) + VisEdgeA3(1)*(Pre_dis^3) - dy_pre)/sqrt(CuratureDop_pre^2+single(1));
dyRiRE = (VisEdgeA0(2) + VisEdgeA1(2)*Pre_dis + VisEdgeA2(2)*(Pre_dis^2) + VisEdgeA3(2)*(Pre_dis^3) - dy_pre)/sqrt(CuratureDop_pre^2+single(1));

Error = Y_Line-Y_DOP;
Error2= dy_pre - Y_Line;





%%       DOP到车道线切换    
% DoubleLine_Pre2Cent_Dislimit = 1
% DoubleLine_Curr2Cent_Dislimit = 0.5
% DoubleLine_Dop2Cent_Dislimit =0.5

% SingleLine_Cent2Edge_Dislimit =100

% SingleLine_Pre2Cent_Dislimit = 0.5
% SingleLine_Curr2Cent_Dislimit = 0.2
% SingleLine_Dop2Cent_Dislimit =0.2

if DOP_OUT==1&&Line_State~=0
     DOP2Cent_flag = uint8(1);
elseif DOP_OUT==0
    if Line_State~=1 && Line_State~=2 && Line_State~=0 
        if (abs(Error2)<DoubleLine_Pre2Cent_Dislimit || abs(CentLineA0)<DoubleLine_Curr2Cent_Dislimit || abs(Error)< DoubleLine_Dop2Cent_Dislimit)&&...
                abs(CentLineA1)<DoubleLine_DOPOut_C1
            DOP2Cent_flag = uint8(1);
        end
    else
        if Line_State~=0 
%             if ((VisEdgeConf(1)>=1 && abs(abs(dyLeRE-Y_Line)-abs(VisEdgeA0(1)-CentLineA0))<SingleLine_Cent2Edge_Dislimit)||...
%                     (VisEdgeConf(2)>=1 && abs(abs(dyRiRE-Y_Line)-abs(VisEdgeA0(2)-CentLineA0))<SingleLine_Cent2Edge_Dislimit)) &&...
            if (abs(Error2)<SingleLine_Pre2Cent_Dislimit || abs(CentLineA0)<SingleLine_Curr2Cent_Dislimit || abs(Error)< SingleLine_Dop2Cent_Dislimit)&&...
                    abs(CentLineA1)<SingleLine_DOPOut_C1
                DOP2Cent_flag = uint8(1);
            end
        end

    end
end


%%       OFF到车道线
if  CentLaneValid==true
    Off2Cent_flag=uint8(1);
end
%%       OFF到DOP
if DOP_EN==1 && Vehicle_Speed<55
    Off2DOP_flag=uint8(1);
end
%%       车道线到OFF
if Line_State==0
    Cent2Off_flag=uint8(1);
end
%%       DOP到OFF
if DOP_OUT==1||Vehicle_Speed>=60
    DOP2Off_flag=uint8(1);
end
%%       车道线到DOP
if Line_State==0&&DOP_EN==1&&Vehicle_Speed<55
    Cent2DOP_flag=uint8(1);
end

== matlab function PubIfDecisionLSM_MDL/Subsystem1/TargetLineCalc_20ms/TargetLineCalc/Subsystem5/MATLAB Function3 ==
  data: C12 input; Fac1 output single; C13 input; Fac2 output single; Fac3 output single
function [Fac1,Fac2,Fac3]  = fcn(C12,C13)

C21 = 1/C12;
C31 = 1/C13;

C32 = C12/C13;

C23 = C13/C12;



C = [1,   C12,   C13;
    C21,   1,    C23;
    C31,  C32,    1];

Fac1 = 1/(1 + C21 + C31 );
Fac2 = 1/(C12 + 1+ C32 );
Fac3 = 1/(C13 + C23 + 1 );
